simulink model "Commander_Stabilizer_Qdrone_serial"  (R2019a)
settings: Solver=ode2  StartTime=0.0  StopTime=inf  FixedStep=0.001  RelTol=1e-3  EnableMultiTasking=on
InitFcn:
  | set_param(gcs, 'ZoomFactor','FitSystem')
model workspace (MAT data in the model file):
  target_system = 1
undefined symbols (not defined in the file or in its folder): HIL, qc_get_step_size
libraries: quarc_library x53, simulink x24, simulink_extras x4
(part 4 of 4)

== matlab function Commander_Stabilizer_Qdrone_serial/STABILIZER - QDRONE /PIV CASCADE CONTROLLER1/PID 1/MATLAB Function1 ==
  data: Kp output; Ki output; Kd output
function [Kp, Ki, Kd] = PID_gains()

Kp = 1.3606;%1.2290;
Ki = 0;
Kd = 0.13;%0.1174;

end

== matlab function Commander_Stabilizer_Qdrone_serial/STABILIZER - QDRONE /PHYSICAL PLANT w// NON-LINEAR THRUST/QDrone DAQ/Red - Low Voltage Green - Armed Blue - Disarmed/MATLAB Function LED Color Assignment ==
  data: arm input; value output; low_battery input
function value = fcn(arm, low_battery)

if low_battery
    value = 1;
elseif arm
    value = 2;
else 
    value = 3;
end

== matlab function Commander_Stabilizer_Qdrone_serial/Communication/Detect Communication Loss/MATLAB Function ==
  settings: updateMethod=DISCRETE
  data: time input; stream_connection_loss output; state input; error input; height input; data_loss output; minimum_flight_height input
function [stream_connection_loss , data_loss] = fcn(time, state, error, height, minimum_flight_height)

persistent height_prev
    if isempty(height_prev)
        height_prev = 0;
    end

stream_connection_loss = 0;
data_loss = 0;
if time > 3
    if ((state ~= 2)&&(error < 0))
        % stream connection is not established correctly
        stream_connection_loss = 1;
    end

    if (height == height_prev)&&(height > minimum_flight_height)
        % data is stale
        data_loss = 1;
    end
end

height_prev = height;

== matlab function Commander_Stabilizer_Qdrone_serial/HORIZON FRAME CONVERSION AND ESTIMATION/Calculate Rotation Matrices/MATLAB Function2 ==
  data: roll input; HF_R_BF output; pitch input
function HF_R_BF = rot_xy(roll, pitch)
% Convert from Body Frame to Inertial Frame
% If Yaw = 0, converts from Body Frame to Horizontal Frame instead

Rx  = [1          0           0 ;...
       0  cos(roll)  -sin(roll) ;...
       0  sin(roll)   cos(roll)];
       
Ry  = [cos(pitch)  0  sin(pitch) ;...
                0  1           0 ;...
      -sin(pitch)  0  cos(pitch)];

HF_R_BF = Rx*Ry;

== matlab function Commander_Stabilizer_Qdrone_serial/Pull Detector1/MATLAB Function ==
  settings: updateMethod=DISCRETE  sampleTime=0.001
  data: error_z input; acc_x input; acc_y input; acc_z input; roll input; pitch input; yaw input; detection_output output
function detection_output  = LSTM(error_z, acc_x, acc_y, acc_z, roll, pitch, yaw)

persistent drone_handover_model
persistent p_01_h_t
persistent p_01_c_t
persistent p_03_h_t
persistent p_03_c_t
persistent scaling_params
persistent buffer
persistent counter
persistent clean_detection

downsample_by = 5;

if isempty(drone_handover_model)
    drone_handover_model = coder.load('Model_2f_norm/drone_handover_model.mat');
    scaling_params = coder.load('Model_2f_norm/Scaling.mat');
    p_01_h_t = single(zeros(1,200));
    p_01_c_t = single(randn(1,200)/10);
    p_03_h_t = single(zeros(1,100));
    p_03_c_t = single(randn(1,100)/10);
    buffer = single(zeros(7,downsample_by));
    counter = 1;
    clean_detection = 0;
end

buffer(1,counter) = error_z;
buffer(2,counter) = acc_x;
buffer(3,counter) = acc_y;
buffer(4,counter) = acc_z;
buffer(5,counter) = roll;
buffer(6,counter) = pitch;
buffer(7,counter) = yaw;

if counter == 5
    counter = 1;
    error_z = mean(buffer(1,:));
    acc_x = mean(buffer(2,:));
    acc_y = mean(buffer(3,:));
    acc_z = mean(buffer(4,:));
    roll = mean(buffer(5,:));
    pitch = mean(buffer(6,:));
    yaw = mean(buffer(7,:));
    % 
    [acc_x_inertial, acc_y_inertial, acc_z_inertial] = R_B2I(roll, pitch, yaw, acc_x, acc_y, acc_z);
    % 
    l2_norm_acc_inertial = sqrt(acc_x_inertial.^2 + acc_y_inertial.^2);
    % 
    % [ori_body_x, ori_body_y, ori_body_z] = R_I2B(roll, pitch, yaw, 0, 0, 1);
    % 
%     l2_norm_ori = sqrt(ori_body_x.^2 + ori_body_y.^2);
%     % 
%     acc_dir = atan2(acc_y_inertial, acc_x_inertial);
%     ori_dir = atan2(ori_body_y, ori_body_x);
%     
%     if abs(acc_dir - ori_dir) <= pi
%         dist_acc_ori = abs(acc_dir - ori_dir);
%     else
%         dist_acc_ori = 2*pi - abs(acc_dir - ori_dir);
%     end
    
    % %%Scaling
    % % X_std = (X - X.min(axis=0)) / (X.max(axis=0) - X.min(axis=0))
    error_z = (error_z - scaling_params.data_Z_params(1)) / (scaling_params.data_Z_params(2)-scaling_params.data_Z_params(1));
    error_z = error_z * 2 - 1;
    l2_norm_acc_inertial = (l2_norm_acc_inertial  - scaling_params.data_L2_norm_inertial_params(1)) / (scaling_params.data_L2_norm_inertial_params(2)-scaling_params.data_L2_norm_inertial_params(1));
    l2_norm_acc_inertial = l2_norm_acc_inertial * 2 - 1;
    %     l2_norm_ori = (l2_norm_ori - scaling_params.data_L2_norm_ori_params(1)) / (scaling_params.data_L2_norm_ori_params(2)-scaling_params.data_L2_norm_ori_params(1));
%     dist_acc_ori = (dist_acc_ori - scaling_params.data_dist_acc_ori_params(1)) / (scaling_params.data_dist_acc_ori_params(2)-scaling_params.data_dist_acc_ori_params(1));
    % 

    input_data = [error_z l2_norm_acc_inertial];

    [detection, p_01_c_t, p_01_h_t, p_03_c_t, p_03_h_t] = model_classify(input_data, ...
                                                                         drone_handover_model, ...
                                                                         p_01_c_t, ...
                                                                         p_01_h_t, ...
                                                                         p_03_c_t, ...
                                                                         p_03_h_t);
                                                                     
    clean_detection = clean(detection, 0.5);
%     clean_detection = double(detection);
end

counter = counter + 1;

% dist_acc_ori_out = dist_acc_ori;
% l2_norm_ori_out = l2_norm_ori;
% l2_norm_acc_out = l2_norm_acc_inertial;
detection_output = double(clean_detection);

% function [detection_output, error_output, l2_output] = LSTM_offline(error_z_, l2_norm_acc_inertial_)
% 
% persistent drone_handover_model
% persistent p_01_h_t
% persistent p_01_c_t
% persistent p_03_h_t
% persistent p_03_c_t
% persistent scaling_params
% persistent buffer
% persistent counter
% persistent clean_detection
% 
% downsample_by = 5;
% 
% if isempty(drone_handover_model)
%     drone_handover_model = coder.load('Model_2f_norm/drone_handover_model.mat');
%     p_01_h_t = single(zeros(1,200));
%     p_01_c_t = single(randn(1,200)/10);
%     p_03_h_t = single(zeros(1,100));
%     p_03_c_t = single(randn(1,100)/10);
%     buffer = single(zeros(7,downsample_by));
%     counter = 1;
%     clean_detection = 0;
% end
% 
% 
% input_data = [error_z_ l2_norm_acc_inertial_];
% 
% [detection, p_01_c_t, p_01_h_t, p_03_c_t, p_03_h_t] = model_classify(input_data, ...
%                                                                      drone_handover_model, ...
%                                                                      p_01_c_t, ...
%                                                                      p_01_h_t, ...
%                                                                      p_03_c_t, ...
%                                                                      p_03_h_t);
% 
% clean_detection = clean(detection, 0.5);
% 
% error_output = error_z_;
% l2_output = l2_norm_acc_inertial_;
% detection_output = double(clean_detection);

== matlab function Commander_Stabilizer_Qdrone_serial/HORIZON FRAME CONVERSION AND ESTIMATION/Calculate Rotation Matrices/MATLAB Function4 ==
  data: yaw input; HF_R_IF output
function HF_R_IF = rot_z(yaw)
% Convert from Inertial Frame to Horizontal Frame

HF_R_IF = [cos(yaw)  sin(yaw)  0 ;...
            -sin(yaw)  cos(yaw)  0 ;...
                    0         0  1];

== matlab function Commander_Stabilizer_Qdrone_serial/Pull Detector1/MATLAB Function1 ==
  settings: updateMethod=DISCRETE  sampleTime=0.001
  data: u input; y output; threshold input
function y = prediction_filter(u, threshold)

persistent counter_ones
persistent counter_zeros
persistent pull_detected
persistent prev_u

if isempty(counter_ones)
    counter_ones = 0;
    counter_zeros = 0;
    prev_u = 0;
end

if u == 1
    counter_ones = counter_ones + 1;
else
    counter_zeros = counter_zeros + 1;     
end

if prev_u == 0 && u == 1
    counter_zeros = 0;
end

if counter_ones > threshold && counter_zeros < threshold
    pull_detected = 1;
else
    pull_detected = 0;
end

if counter_zeros >= threshold
    counter_ones = 0;
end

prev_u = double(u);
y = pull_detected;

== matlab function Commander_Stabilizer_Qdrone_serial/STABILIZER - QDRONE /PIV CASCADE CONTROLLER1/MRFT_NEW /MATLAB Function ==
  settings: updateMethod=DISCRETE
  data: err input; output output; beta input; h input; no_switch_delay_in_s input; num_of_peak_conf_samples input; sim_time input; e_max_o output; e_min_o output; sw_max_o output; sw_min_o output
% MRFT algorithm with false switching prevention mechanism
% June 2020
% Coded By M. Chehadeh, Khalifa University
function [output,e_max_o,e_min_o,sw_max_o,sw_min_o]  = MRFT(err,beta,h,no_switch_delay_in_s,num_of_peak_conf_samples,sim_time)
persistent switch_time;
persistent last_output;
persistent e_max;
persistent e_min;
persistent has_reached_min;
persistent has_reached_max;
persistent peak_conf_counter;
mode_of_operation=1;
% mode_of_operation=0 take last e_max or e_min
% mode_of_operation=1 take current e_max or e_min and mirror it

output=0;
e_max_o=0;
e_min_o=0;
sw_max_o=0;
sw_min_o=0;
if isempty(switch_time)
    switch_time = sim_time;
    peak_conf_counter=0;
    e_max=0;
    e_min=0;
    if (err>0)
        has_reached_max=true;
        has_reached_min=false;
        last_output=h;
    else
        has_reached_max=false;
        has_reached_min=true;
        last_output=-h;
    end
    output=last_output;
    return;  
end
output=last_output;
if (sim_time-switch_time<=no_switch_delay_in_s)
    e_min_o=e_min;
    e_max_o=e_max;
    return;
end

if (last_output<0)
    if (err<e_min)
        e_min=err;
        peak_conf_counter=0;
    else
        peak_conf_counter=peak_conf_counter+1;
        if (peak_conf_counter>=num_of_peak_conf_samples)
            has_reached_min=true;
            peak_conf_counter=0;
        end
        e_max=err;
    end
    if (mode_of_operation==0)
        sw_min=((e_max-e_min)/2)+e_min+beta*((e_max-e_min)/2);
    elseif (mode_of_operation==1)
        e_max_star=-e_min;
        sw_min=((e_max_star-e_min)/2)+e_min+beta*((e_max_star-e_min)/2);
    end
    sw_min_o=sw_min;
    if (has_reached_min)
        if (err>sw_min)
            output=h;
            switch_time=sim_time;
            has_reached_min=false;
        else
            output=last_output;
        end
    end
else
    if (err>e_max)
        e_max=err;
        peak_conf_counter=0;
    else
        peak_conf_counter=peak_conf_counter+1;
        if (peak_conf_counter>=num_of_peak_conf_samples)
            has_reached_max=true;
            peak_conf_counter=0;
        end
        e_min=err;
    end
    if (mode_of_operation==0)
        sw_max=e_max-((e_max-e_min)/2)-(beta*((e_max-e_min)/2));
    elseif (mode_of_operation==1)
        e_min_star=-e_max;
        sw_max=e_max-((e_max-e_min_star)/2)-(beta*((e_max-e_min_star)/2));
    end    
    sw_max_o=sw_max;
    if (has_reached_max)
        if (err<sw_max)
            output=-h;
            switch_time=sim_time;
            has_reached_max=false;
        else
            output=last_output;
        end
    end
end
e_min_o=e_min;
e_max_o=e_max;
last_output=output;

== matlab function Commander_Stabilizer_Qdrone_serial/STABILIZER - QDRONE /PIV CASCADE CONTROLLER1/MRFT_NEW 1/MATLAB Function ==
  settings: updateMethod=DISCRETE
  data: err input; output output; beta input; h input; no_switch_delay_in_s input; num_of_peak_conf_samples input; sim_time input; e_max_o output; e_min_o output; sw_max_o output; sw_min_o output
% MRFT algorithm with false switching prevention mechanism
% June 2020
% Coded By M. Chehadeh, Khalifa University
function [output,e_max_o,e_min_o,sw_max_o,sw_min_o]  = MRFT(err,beta,h,no_switch_delay_in_s,num_of_peak_conf_samples,sim_time)
persistent switch_time;
persistent last_output;
persistent e_max;
persistent e_min;
persistent has_reached_min;
persistent has_reached_max;
persistent peak_conf_counter;
mode_of_operation=1;
% mode_of_operation=0 take last e_max or e_min
% mode_of_operation=1 take current e_max or e_min and mirror it

output=0;
e_max_o=0;
e_min_o=0;
sw_max_o=0;
sw_min_o=0;
if isempty(switch_time)
    switch_time = sim_time;
    peak_conf_counter=0;
    e_max=0;
    e_min=0;
    if (err>0)
        has_reached_max=true;
        has_reached_min=false;
        last_output=h;
    else
        has_reached_max=false;
        has_reached_min=true;
        last_output=-h;
    end
    output=last_output;
    return;  
end
output=last_output;
if (sim_time-switch_time<=no_switch_delay_in_s)
    e_min_o=e_min;
    e_max_o=e_max;
    return;
end

if (last_output<0)
    if (err<e_min)
        e_min=err;
        peak_conf_counter=0;
    else
        peak_conf_counter=peak_conf_counter+1;
        if (peak_conf_counter>=num_of_peak_conf_samples)
            has_reached_min=true;
            peak_conf_counter=0;
        end
        e_max=err;
    end
    if (mode_of_operation==0)
        sw_min=((e_max-e_min)/2)+e_min+beta*((e_max-e_min)/2);
    elseif (mode_of_operation==1)
        e_max_star=-e_min;
        sw_min=((e_max_star-e_min)/2)+e_min+beta*((e_max_star-e_min)/2);
    end
    sw_min_o=sw_min;
    if (has_reached_min)
        if (err>sw_min)
            output=h;
            switch_time=sim_time;
            has_reached_min=false;
        else
            output=last_output;
        end
    end
else
    if (err>e_max)
        e_max=err;
        peak_conf_counter=0;
    else
        peak_conf_counter=peak_conf_counter+1;
        if (peak_conf_counter>=num_of_peak_conf_samples)
            has_reached_max=true;
            peak_conf_counter=0;
        end
        e_min=err;
    end
    if (mode_of_operation==0)
        sw_max=e_max-((e_max-e_min)/2)-(beta*((e_max-e_min)/2));
    elseif (mode_of_operation==1)
        e_min_star=-e_max;
        sw_max=e_max-((e_max-e_min_star)/2)-(beta*((e_max-e_min_star)/2));
    end    
    sw_max_o=sw_max;
    if (has_reached_max)
        if (err<sw_max)
            output=-h;
            switch_time=sim_time;
            has_reached_max=false;
        else
            output=last_output;
        end
    end
end
e_min_o=e_min;
e_max_o=e_max;
last_output=output;

== matlab function Commander_Stabilizer_Qdrone_serial/STABILIZER - QDRONE /PIV CASCADE CONTROLLER1/Body frame attitude error1 ==
  data: roll_ref input; pitch_ref input; yaw_ref input; e_roll output; e_pitch output; e_yaw output; DCM input
function [e_roll, e_pitch, e_yaw] = fcn(roll_ref, pitch_ref, yaw_ref, DCM)

DCM_yaw_ref = [cos(yaw_ref), -sin(yaw_ref), 0;
                sin(yaw_ref), cos(yaw_ref), 0;
                0, 0, 1];

yaw_ref = 0;
theta_ref = norm([roll_ref, pitch_ref, yaw_ref]);

if(theta_ref ~= 0)
    euler_axis_ref = [roll_ref, pitch_ref, yaw_ref] / theta_ref;
else
    euler_axis_ref = [0, 0, 0];
end

%limit theta_ref
theta_ref = min(pi/2, max(theta_ref, -pi/2));

quaternion_ref = euler_axis_ref * sin(theta_ref / 2);
quaternion_ref = [cos(theta_ref / 2), quaternion_ref];

DCM_ref = DCM_yaw_ref * quat2rotm(quaternion_ref);

DCM_error = transpose(DCM) * DCM_ref;

g = trace((trace(DCM_error) - 1) / 2);
g = min(1, max(g, -1));
theta_error = acos(g);

if(theta_error ~= 0)
    e_roll = theta_error * ( DCM_error(3,2) - DCM_error(2,3) ) / (2 * sin(theta_error));
    e_pitch = theta_error * ( DCM_error(1,3) - DCM_error(3,1) ) / (2 * sin(theta_error));
    e_yaw = theta_error * ( DCM_error(2,1) - DCM_error(1,2) ) / (2 * sin(theta_error));
else
    e_roll = 0;
    e_pitch = 0;
    e_yaw = 0;
end


end

== matlab function Commander_Stabilizer_Qdrone_serial/STABILIZER - QDRONE /PIV CASCADE CONTROLLER1/DCM constructor  ==
  data: roll input; DCM output; pitch input; yaw input
function DCM = fcn(roll, pitch, yaw)

%DCM of yaw
yaw_DCM = [cos(yaw) -sin(yaw) 0;
            sin(yaw) cos(yaw) 0;
            0 0 1];
        
% pitch_DCM = [cos(pitch) 0 sin(pitch);
%             0, 1, 0;
%             -sin(pitch) 0 cos(pitch)];
%         
% roll_DCM = [1, 0, 0;
%             0 cos(yaw) -sin(roll);
%             0 sin(roll) cos(roll)];
%      
% DCM = yaw_DCM * pitch_DCM * roll_DCM;


% DCM of roll/pitch
theta_err = norm([roll, pitch, 0]);
euler_axis_err = [0, 0, 0];
if(theta_err ~= 0)
    euler_axis_err = [roll, pitch, 0] / theta_err;
end
%limit theta_ref
theta_err = min(pi/2, max(theta_err, -pi/2));
quaternion_err = euler_axis_err * sin(theta_err / 2);
quaternion_err = [cos(theta_err / 2), quaternion_err];
roll_pitch_DCM = quat2rotm(quaternion_err);


DCM = yaw_DCM * roll_pitch_DCM;

end

== matlab function Commander_Stabilizer_Qdrone_serial/STABILIZER - QDRONE /PIV CASCADE CONTROLLER1/PID yaw/MATLAB Function1 ==
  data: Kp output; Ki output; Kd output
function [Kp, Ki, Kd] = PID_gains()

Kp = 0.6;
Ki = 0;
Kd = 0.12;

end

== matlab function Commander_Stabilizer_Qdrone_serial/STABILIZER - QDRONE /PIV CASCADE CONTROLLER1/throttle limiter ==
  data: throttle_in input; e_roll input; e_pitch input; e_yaw input; throttle_out output
function throttle_out = fcn(throttle_in, e_roll, e_pitch, e_yaw)

throttle_out = throttle_in * cos(norm([e_roll, e_pitch, e_yaw]));

if (throttle_out < 0) 
    throttle_out = 0;
end
